simulink model "EHB_MOTOR0313"  (R2022a)
settings: Solver=FixedStepAuto  StartTime=0.0  StopTime=10  FixedStep=0.0001  RelTol=1e-3  EnableMultiTasking=on
undefined symbols (not defined in the file): Cos_Table, Cos_Table1, Sin_BreakPoint, Sin_BreakPoint1, Sin_Table, Sin_Table1
libraries: simulink x7
(part 2 of 2)

== system EHB_MOTOR0313/EHB_MOTOR_PRO/Function-Call Subsystem1/Current_Transform/Ia_caculate/Subsystem1 ==
  Ib_Inte : Inport  OutDataTypeStr=uint16
  Add1 : Sum  Inputs=+-  OutDataTypeStr=int16
  Constant4 : Constant  Value=2042  OutDataTypeStr=int16
  Gain3 : Gain  Gain=0.0814  OutDataTypeStr=single
  V : Outport
  wires:
  Add1/1 -> Gain3/1
  Gain3/1 -> V/1
  Ib_Inte/1 -> Add1/1
  Constant4/1 -> Add1/2

== system EHB_MOTOR0313/EHB_MOTOR_PRO/Function-Call Subsystem1/Current_Transform/Ia_caculate/Subsystem2 ==
  Ic_Inte : Inport  OutDataTypeStr=uint16
  Add2 : Sum  Inputs=+-  OutDataTypeStr=int16
  Constant6 : Constant  Value=2041  OutDataTypeStr=int16
  Gain7 : Gain  Gain=0.0814  OutDataTypeStr=single
  W : Outport
  wires:
  Gain7/1 -> W/1
  Ic_Inte/1 -> Add2/1
  Constant6/1 -> Add2/2
  Add2/1 -> Gain7/1

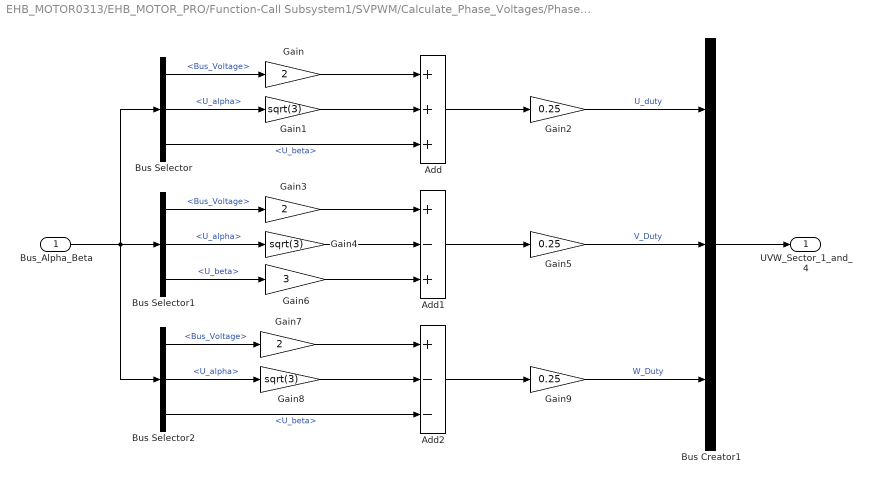
== system EHB_MOTOR0313/EHB_MOTOR_PRO/Function-Call Subsystem1/SVPWM/Calculate_Phase_Voltages/Phase_Voltage_Sectors_1_and_4 ==
  Bus_Alpha_Beta : Inport
  Add : Sum  Inputs=+++
  Add1 : Sum  Inputs=+-+
  Add2 : Sum  Inputs=+--
  Bus Creator1 : BusCreator  Inputs=3
  Bus Selector : BusSelector  OutputSignals=Bus_Voltage,U_alpha,U_beta
  Bus Selector1 : BusSelector  OutputSignals=Bus_Voltage,U_alpha,U_beta
  Bus Selector2 : BusSelector  OutputSignals=Bus_Voltage,U_alpha,U_beta
  Gain : Gain  Gain=2  OutDataTypeStr=Inherit: Same as input
  Gain1 : Gain  Gain=sqrt(3)  OutDataTypeStr=Inherit: Same as input
  Gain2 : Gain  Gain=0.25  OutDataTypeStr=Inherit: Same as input
  Gain3 : Gain  Gain=2  OutDataTypeStr=Inherit: Same as input
  Gain4 : Gain  Gain=sqrt(3)  OutDataTypeStr=Inherit: Same as input
  Gain5 : Gain  Gain=0.25  OutDataTypeStr=Inherit: Same as input
  Gain6 : Gain  Gain=3  OutDataTypeStr=Inherit: Same as input
  Gain7 : Gain  Gain=2  OutDataTypeStr=Inherit: Same as input
  Gain8 : Gain  Gain=sqrt(3)  OutDataTypeStr=Inherit: Same as input
  Gain9 : Gain  Gain=0.25  OutDataTypeStr=Inherit: Same as input
  UVW_Sector_1_and_4 : Outport  OutDataTypeStr=single  VectorParamsAs1DForOutWhenUnconnected=off
  wires:
  Gain2/1 -> Bus Creator1/1  "U_duty"
  Bus Selector/1 -> Gain/1  "<Bus_Voltage>"
  Bus Selector/3 -> Add/3  "<U_beta>"
  Gain/1 -> Add/1
  Add/1 -> Gain2/1
  Gain1/1 -> Add/2
  Bus Selector/2 -> Gain1/1  "<U_alpha>"
  Gain6/1 -> Add1/3
  Gain4/1 -> Add1/2
  Bus Selector1/3 -> Gain6/1  "<U_beta>"
  Gain3/1 -> Add1/1
  Add1/1 -> Gain5/1
  Bus Selector1/1 -> Gain3/1  "<Bus_Voltage>"
  Gain5/1 -> Bus Creator1/2  "V_Duty"
  Bus Selector1/2 -> Gain4/1  "<U_alpha>"
  Add2/1 -> Gain9/1
  Gain8/1 -> Add2/2
  Gain7/1 -> Add2/1
  Bus_Alpha_Beta/1 -> Bus Selector2/1, Bus Selector/1, Bus Selector1/1
  Bus Selector2/2 -> Gain8/1  "<U_alpha>"
  Bus Selector2/3 -> Add2/3  "<U_beta>"
  Gain9/1 -> Bus Creator1/3  "W_Duty"
  Bus Selector2/1 -> Gain7/1  "<Bus_Voltage>"
  Bus Creator1/1 -> UVW_Sector_1_and_4/1

== system EHB_MOTOR0313/EHB_MOTOR_PRO/Function-Call Subsystem1/SVPWM/Calculate_Phase_Voltages/U_Sectors_2_and_5 ==
  Bus_Alpha : Inport
  Add : Sum
  Add1 : Sum  OutDataTypeStr=single
  Add2 : Sum  Inputs=+-
  Bus Creator2 : BusCreator  Inputs=3
  Bus Selector : BusSelector  OutputSignals=Bus_Voltage,U_alpha
  Bus Selector1 : BusSelector  OutputSignals=Bus_Voltage,U_beta
  Bus Selector2 : BusSelector  OutputSignals=Bus_Voltage,U_beta
  Gain1 : Gain  Gain=sqrt(3)  OutDataTypeStr=Inherit: Same as input
  Gain2 : Gain  Gain=0.5  OutDataTypeStr=Inherit: Same as input
  Gain3 : Gain  Gain=0.5  OutDataTypeStr=single
  Gain4 : Gain  Gain=0.5  OutDataTypeStr=Inherit: Same as input
  UVW_Sector_2_and_5 : Outport  VectorParamsAs1DForOutWhenUnconnected=off
  wires:
  Bus Selector/2 -> Gain1/1  "<U_alpha>"
  Gain1/1 -> Add/2
  Add/1 -> Gain2/1
  Bus Selector/1 -> Add/1  "<Bus_Voltage>"
  Bus Selector1/1 -> Add1/1  "<Bus_Voltage>"
  Bus_Alpha/1 -> Bus Selector2/1, Bus Selector1/1, Bus Selector/1  "Bus_Beta"
  Bus Selector1/2 -> Add1/2  "<U_beta>"
  Add1/1 -> Gain3/1
  Add2/1 -> Gain4/1
  Bus Selector2/1 -> Add2/1  "<Bus_Voltage>"
  Gain4/1 -> Bus Creator2/3
  Bus Selector2/2 -> Add2/2  "<U_beta>"
  Gain2/1 -> Bus Creator2/1
  Gain3/1 -> Bus Creator2/2
  Bus Creator2/1 -> UVW_Sector_2_and_5/1

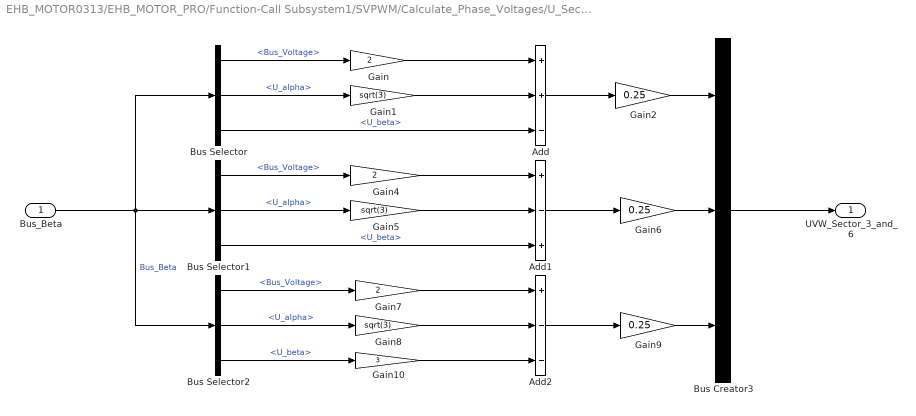
== system EHB_MOTOR0313/EHB_MOTOR_PRO/Function-Call Subsystem1/SVPWM/Calculate_Phase_Voltages/U_Sectors_3_and_6 ==
  Bus_Beta : Inport
  Add : Sum  Inputs=++-  OutDataTypeStr=single
  Add1 : Sum  Inputs=+-+  OutDataTypeStr=single
  Add2 : Sum  Inputs=+--  OutDataTypeStr=single
  Bus Creator3 : BusCreator  Inputs=3
  Bus Selector : BusSelector  OutputSignals=Bus_Voltage,U_alpha,U_beta
  Bus Selector1 : BusSelector  OutputSignals=Bus_Voltage,U_alpha,U_beta
  Bus Selector2 : BusSelector  OutputSignals=Bus_Voltage,U_alpha,U_beta
  Gain : Gain  Gain=2  OutDataTypeStr=Inherit: Same as input
  Gain1 : Gain  Gain=sqrt(3)  OutDataTypeStr=Inherit: Same as input
  Gain10 : Gain  Gain=3  OutDataTypeStr=single
  Gain2 : Gain  Gain=0.25  OutDataTypeStr=Inherit: Same as input
  Gain4 : Gain  Gain=2  OutDataTypeStr=Inherit: Same as input
  Gain5 : Gain  Gain=sqrt(3)  OutDataTypeStr=Inherit: Same as input
  Gain6 : Gain  Gain=0.25  OutDataTypeStr=Inherit: Same as input
  Gain7 : Gain  Gain=2  OutDataTypeStr=Inherit: Same as input
  Gain8 : Gain  Gain=sqrt(3)  OutDataTypeStr=Inherit: Same as input
  Gain9 : Gain  Gain=0.25  OutDataTypeStr=Inherit: Same as input
  UVW_Sector_3_and_6 : Outport  VectorParamsAs1DForOutWhenUnconnected=off
  wires:
  Bus Selector/1 -> Gain/1  "<Bus_Voltage>"
  Add/1 -> Gain2/1
  Bus Selector/3 -> Add/3  "<U_beta>"
  Gain/1 -> Add/1
  Gain1/1 -> Add/2
  Bus Selector/2 -> Gain1/1  "<U_alpha>"
  Bus Selector1/1 -> Gain4/1  "<Bus_Voltage>"
  Bus Selector1/2 -> Gain5/1  "<U_alpha>"
  Gain5/1 -> Add1/2
  Gain4/1 -> Add1/1
  Bus_Beta/1 -> Bus Selector2/1, Bus Selector1/1, Bus Selector/1  "Bus_Beta"
  Bus Selector1/3 -> Add1/3  "<U_beta>"
  Add1/1 -> Gain6/1
  Bus Selector2/2 -> Gain8/1  "<U_alpha>"
  Gain7/1 -> Add2/1
  Gain10/1 -> Add2/3
  Gain8/1 -> Add2/2
  Add2/1 -> Gain9/1
  Bus Selector2/3 -> Gain10/1  "<U_beta>"
  Bus Selector2/1 -> Gain7/1  "<Bus_Voltage>"
  Gain2/1 -> Bus Creator3/1
  Gain6/1 -> Bus Creator3/2
  Gain9/1 -> Bus Creator3/3
  Bus Creator3/1 -> UVW_Sector_3_and_6/1
